simulink model "chooseTapB"  (Simulink 7.6)
settings: Solver=ode45  StartTime=0.0  StopTime=0.3  RelTol=1e-3
PreLoadFcn:
  | init
libraries: powerlib x19, dspsnks4 x5, fuzblock x3, factslib x1, powerlib_extras x1
settings Model: Creator=chix  LastModifiedBy=chix

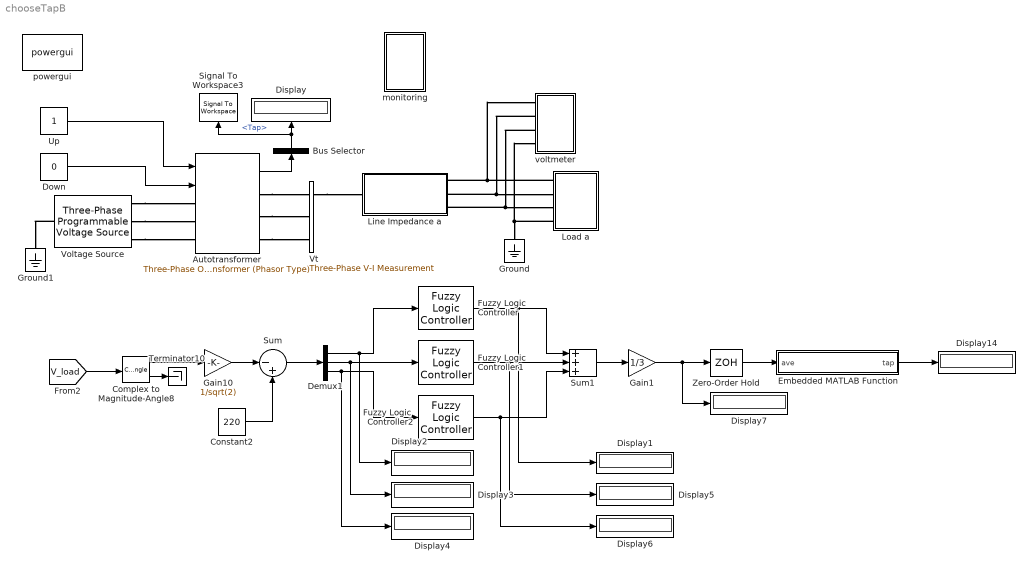
== system chooseTapB ==
  Autotransformer : factslib/Transformers/Three-Phase OLTC Regulating Transformer (Phasor Type)  DialogController=POWERSYS.PowerSysDialog  SystemSampleTime=-1  ShowParam=OLTC and Voltage Regulator parameters  PnomFnom="[200  60]"  Winding1=[220*sqrt(3) 0.00171 0.01714 ]  Winding1Connection=Yg  Winding2="[215*sqrt(3)   0.00094 0.01654 ]"  Winding2Connection=Yg  WindingTap=[ 0.00187 0.00142]  RmXm=[18.16805 1040.85906]  TapOnWinding=Winding 2  dU=3/215  TapMinMax="[ 0  4]"  InitialTap=2  TapSelectionTime=0.001  ExternalControl=on  RegulatorOn=on  Regulator=[1.0233 0.007 1]  Iw2_init="[0   0]"
  Bus Selector : BusSelector  OutputSignals=Tap
  Complex to Magnitude-Angle8 : ComplexToMagnitudeAngle
  Constant2 : Constant  Value=220
  Demux1 : Demux  Outputs=3
  Display{,1..7,14} (9 alike) : Display
  Down : Constant  Value=0
  Embedded MATLAB Function : Stateflow chart  TreatAsAtomicUnit=on
  Fuzzy Logic  Controller : fuzblock/Fuzzy Logic  Controller  SystemSampleTime=-1  fis='dataGather_w_con_1input_1.fis'
  Fuzzy Logic  Controller1 : fuzblock/Fuzzy Logic  Controller  SystemSampleTime=-1  fis='dataGather_w_con_1input_2.fis'
  Fuzzy Logic  Controller2 : fuzblock/Fuzzy Logic  Controller  SystemSampleTime=-1  fis='dataGather_w_con_1input_3.fis'
  Gain1 : Gain  Gain=1/3
  Gain10 : Gain  Gain=1/sqrt(2)
  Ground : powerlib/Elements/Ground  DialogController=POWERSYS.PowerSysDialog  PhysicalDomain=powersysdomain  SubClassName=unknown  LeftPortType=p1  RightPortType=p1  LConnTagsString=a
  Ground1 : powerlib/Elements/Ground  DialogController=POWERSYS.PowerSysDialog  PhysicalDomain=powersysdomain  SubClassName=unknown  LeftPortType=p1  RightPortType=p1  LConnTagsString=a
  Line Impedance a : Subsystem
  Load a : Subsystem
  Signal To Workspace3 : dspsnks4/Signal To Workspace  SystemSampleTime=-1  VariableName=tap  FrameMode=Concatenate frames (2-D array)
      settings: MaxDataPoints=1  FixptAsFi=off
  Sum : Sum  Inputs=|-+
  Sum1 : Sum  Inputs=+++
  Terminator10 : Terminator
  Up : Constant
  Voltage Source : powerlib/Electrical Sources/Three-Phase Programmable Voltage Source  DialogController=POWERSYS.PowerSysDialog  SystemSampleTime=-1  PositiveSequence="[220*sqrt(3)  0 60]"  VariationEntity=None  VariationType=Step  VariationStep=0.5  VariationRate=10  VariationMagnitude=0.3  VariationFrequency=2  VariationTiming=[1 2]  VariationPhaseA=off  Amplitudes=[1 0.8 1.2 1.0]  TimeValues=[0 0.1 0.15 0.2]  HarmonicGeneration=off  HarmonicA=[3 0.2 -25 0]  HarmonicB=[2 0.15 35 2]  Timing="[0.05  3]"
  Vt : powerlib/Measurements/Three-Phase V-I Measurement  DialogController=POWERSYS.PowerSysDialog  SystemSampleTime=-1  VoltageMeasurement=phase-to-ground  SetLabelV=on  LabelV=Vabc_xmer  Vpu=off  VpuLL=off  CurrentMeasurement=no  SetLabelI=off  LabelI=Iabc  Ipu=off  Pbase=100e6  Vbase=220  OutputType=Magnitude  PhasorSimulation=on  PSBequivalent=0
  Zero-Order Hold : ZeroOrderHold  SampleTime=0.011
  monitoring : Subsystem
  powergui : powerlib/powergui  Priority=1  SystemSampleTime=-1  SimulationMode=Phasor  SampleTime=50e-6  frequency=60  SPID=off  DisableSnubberDevices=off  DisableRonSwitches=off  DisableVfSwitches=off  SwTol=0  Interpol=off  frequencyindice=60  echomessages=off  HookPort=off  DisplayEquations=off  FunctionMessages=off  EnableUseOfTLC=off  x0status=blocks  RestoreLinks=warning  ResistiveCurrentMeasurement=off  Ylog=off  Xlog=on  ShowGrid=off  save=off  variable=ZData  ZoomFFT=off  StartTime=0.0  cycles=1  DisplayStyle=1  FreqAxis=off  MaxFrequency=1000  frequencyindicesteady=1  display=off  methode=off
  voltmeter : Subsystem
  wires:
  Bus Selector/1 -> Display/1, Signal To Workspace3/1  "<Tap>"
  Autotransformer/1 -> Bus Selector/1
  Complex to Magnitude-Angle8/1 -> Gain10/1
  [V_load] -> Complex to Magnitude-Angle8/1
  Gain10/1 -> Sum/1
  Constant2/1 -> Sum/2
  Sum/1 -> Demux1/1
  Demux1/1 -> Display2/1, Fuzzy Logic  Controller/1
  Demux1/3 -> Display4/1, Fuzzy Logic  Controller2/1
  Complex to Magnitude-Angle8/2 -> Terminator10/1
  Demux1/2 -> Display3/1, Fuzzy Logic  Controller1/1
  Fuzzy Logic  Controller/1 -> Display1/1, Sum1/1
  Fuzzy Logic  Controller1/1 -> Display5/1, Sum1/2
  Fuzzy Logic  Controller2/1 -> Display6/1, Sum1/3
  Sum1/1 -> Gain1/1
  Zero-Order Hold/1 -> Embedded MATLAB Function/1(ave)
  Embedded MATLAB Function/1(tap) -> Display14/1
  Gain1/1 -> Zero-Order Hold/1, Display7/1
  Down/1 -> Autotransformer/2
  Up/1 -> Autotransformer/1
  connections:
  Voltage Source/LConn1 -- Ground1/LConn1
  Voltage Source/RConn1 -- Autotransformer/LConn1
  Voltage Source/RConn2 -- Autotransformer/LConn2
  Voltage Source/RConn3 -- Autotransformer/LConn3
  Autotransformer/RConn3 -- Vt/LConn3
  Autotransformer/RConn2 -- Vt/LConn2
  Autotransformer/RConn1 -- Vt/LConn1
  Vt/RConn1 -- Line Impedance a/LConn1
  Load a/LConn4 -- Ground/LConn1 -- voltmeter/LConn4
  voltmeter/LConn3 -- Line Impedance a/RConn3 -- Load a/LConn3
  voltmeter/LConn2 -- Line Impedance a/RConn2 -- Load a/LConn2
  Load a/LConn1 -- Line Impedance a/RConn1 -- voltmeter/LConn1

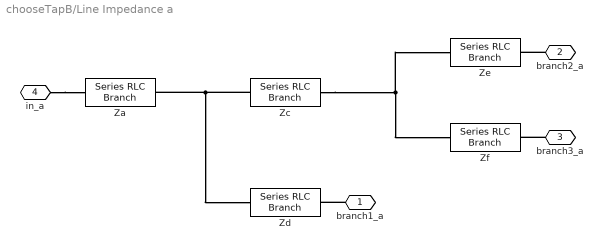
== system chooseTapB/Line Impedance a ==
  Za : powerlib/Elements/Series RLC Branch  DialogController=POWERSYS.PowerSysDialog  PhysicalDomain=powersysdomain  SubClassName=unknown  LeftPortType=p1  RightPortType=p1  LConnTagsString=__new0  RConnTagsString=__new0  BranchType=RL  Resistance=0.014  Inductance=0.0113e-3  SetiL0=off  InitialCurrent=0  Capacitance=1e-6  Setx0=off  InitialVoltage=0  Measurements=None
  Zc : powerlib/Elements/Series RLC Branch  DialogController=POWERSYS.PowerSysDialog  PhysicalDomain=powersysdomain  SubClassName=unknown  LeftPortType=p1  RightPortType=p1  LConnTagsString=__new0  RConnTagsString=__new0  BranchType=RL  Resistance=0.013  Inductance=0.0102e-3  SetiL0=off  InitialCurrent=0  Capacitance=1e-6  Setx0=off  InitialVoltage=0  Measurements=None
  Zd : powerlib/Elements/Series RLC Branch  DialogController=POWERSYS.PowerSysDialog  PhysicalDomain=powersysdomain  SubClassName=unknown  LeftPortType=p1  RightPortType=p1  LConnTagsString=__new0  RConnTagsString=__new0  BranchType=RL  Resistance=11  Inductance=47e-3  SetiL0=off  InitialCurrent=0  Capacitance=1e-6  Setx0=off  InitialVoltage=0  Measurements=None
  Ze : powerlib/Elements/Series RLC Branch  DialogController=POWERSYS.PowerSysDialog  PhysicalDomain=powersysdomain  SubClassName=unknown  LeftPortType=p1  RightPortType=p1  LConnTagsString=__new0  RConnTagsString=__new0  BranchType=RL  Resistance=1  Inductance=47e-3  SetiL0=off  InitialCurrent=0  Capacitance=1e-6  Setx0=off  InitialVoltage=0  Measurements=None
  Zf : powerlib/Elements/Series RLC Branch  DialogController=POWERSYS.PowerSysDialog  PhysicalDomain=powersysdomain  SubClassName=unknown  LeftPortType=p1  RightPortType=p1  LConnTagsString=__new0  RConnTagsString=__new0  BranchType=RL  Resistance=4.7  Inductance=21.5e-3  SetiL0=off  InitialCurrent=0  Capacitance=1e-6  Setx0=off  InitialVoltage=0  Measurements=None
  branch1_a : PMIOPort  Port=1  Side=Right
  branch2_a : PMIOPort  Port=2  Side=Right
  branch3_a : PMIOPort  Port=3  Side=Right
  in_a : PMIOPort  Port=4  Side=Left
  connections:
  Za/RConn1 -- Zc/LConn1 -- Zd/LConn1
  Zc/RConn1 -- Ze/LConn1 -- Zf/LConn1
  branch2_a/RConn1 -- Ze/RConn1
  in_a/RConn1 -- Za/LConn1
  branch3_a/RConn1 -- Zf/RConn1
  branch1_a/RConn1 -- Zd/RConn1

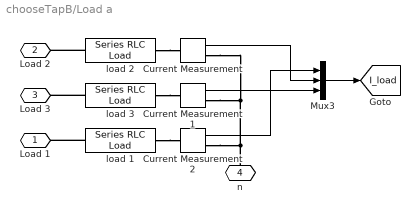
== system chooseTapB/Load a ==
  Current Measurement : powerlib/Measurements/Current Measurement  DialogController=POWERSYS.PowerSysDialog  SystemSampleTime=-1  PhasorSimulation=on  OutputType=Complex  PSBequivalent=0
  Current Measurement1 : powerlib/Measurements/Current Measurement  DialogController=POWERSYS.PowerSysDialog  SystemSampleTime=-1  PhasorSimulation=on  OutputType=Complex  PSBequivalent=0
  Current Measurement2 : powerlib/Measurements/Current Measurement  DialogController=POWERSYS.PowerSysDialog  SystemSampleTime=-1  PhasorSimulation=on  OutputType=Complex  PSBequivalent=0
  Mux3 : Mux  Inputs=3
  load 1 : powerlib/Elements/Series RLC Load  DialogController=POWERSYS.PowerSysDialog  PhysicalDomain=powersysdomain  SubClassName=unknown  LeftPortType=p1  RightPortType=p1  LConnTagsString=a  RConnTagsString=__new0  NominalVoltage=220  NominalFrequency=60  ActivePower=pow1  InductivePower=ql1  CapacitivePower=qc1  Setx0=off  InitialVoltage=0  SetiL0=off  InitialCurrent=0  Measurements=None
  load 2 : powerlib/Elements/Series RLC Load  DialogController=POWERSYS.PowerSysDialog  PhysicalDomain=powersysdomain  SubClassName=unknown  LeftPortType=p1  RightPortType=p1  LConnTagsString=a  RConnTagsString=__new0  NominalVoltage=220  NominalFrequency=60  ActivePower=pow2  InductivePower=ql2  CapacitivePower=qc2  Setx0=off  InitialVoltage=0  SetiL0=off  InitialCurrent=0  Measurements=None
  load 3 : powerlib/Elements/Series RLC Load  DialogController=POWERSYS.PowerSysDialog  PhysicalDomain=powersysdomain  SubClassName=unknown  LeftPortType=p1  RightPortType=p1  LConnTagsString=a  RConnTagsString=__new0  NominalVoltage=220  NominalFrequency=60  ActivePower=pow3  InductivePower=ql3  CapacitivePower=qc3  Setx0=off  InitialVoltage=0  SetiL0=off  InitialCurrent=0  Measurements=None
  Load 1 : PMIOPort  Port=1  Side=Left
  Load 2 : PMIOPort  Port=2  Side=Left
  Load 3 : PMIOPort  Port=3  Side=Left
  n : PMIOPort  Port=4  Side=Left
  tag scope: I_load=global
  wires:
  Mux3/1 -> [I_load]
  Current Measurement/1 -> Mux3/2
  Current Measurement1/1 -> Mux3/3
  Current Measurement2/1 -> Mux3/1
  connections:
  load 2/LConn1 -- Load 2/RConn1
  load 3/LConn1 -- Load 3/RConn1
  load 1/LConn1 -- Load 1/RConn1
  load 2/RConn1 -- Current Measurement/LConn1
  load 3/RConn1 -- Current Measurement1/LConn1
  load 1/RConn1 -- Current Measurement2/LConn1
  n/RConn1 -- Current Measurement/RConn1 -- Current Measurement1/RConn1 -- Current Measurement2/RConn1

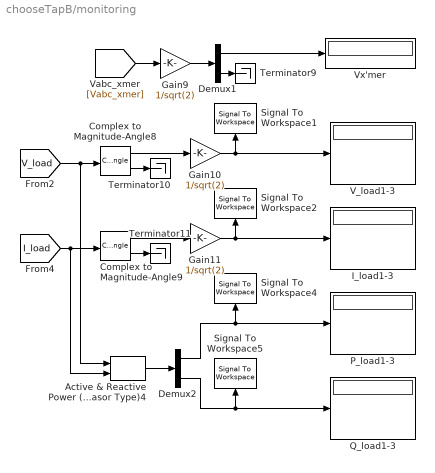
== system chooseTapB/monitoring ==
  Active & Reactive Power (Phasor Type)4 : powerlib_extras/Phasor Library/Active & Reactive Power (Phasor Type)  DialogController=POWERSYS.PowerSysDialog  SystemSampleTime=-1
  Complex to Magnitude-Angle8 : ComplexToMagnitudeAngle
  Complex to Magnitude-Angle9 : ComplexToMagnitudeAngle
  Demux1 : Demux  Outputs=[1 2]
  Demux2 : Demux  Outputs=[3 3]
  Gain10 : Gain  Gain=1/sqrt(2)
  Gain11 : Gain  Gain=1/sqrt(2)
  Gain9 : Gain  Gain=1/sqrt(2)
  I_load1-3 : Display
  P_load1-3 : Display
  Q_load1-3 : Display
  Signal To Workspace1 : dspsnks4/Signal To Workspace  SystemSampleTime=-1  VariableName=vload  FrameMode=Concatenate frames (2-D array)
      settings: MaxDataPoints=1  FixptAsFi=off
  Signal To Workspace2 : dspsnks4/Signal To Workspace  SystemSampleTime=-1  VariableName=iload  FrameMode=Concatenate frames (2-D array)
      settings: MaxDataPoints=1  FixptAsFi=off
  Signal To Workspace4 : dspsnks4/Signal To Workspace  SystemSampleTime=-1  VariableName=pload  FrameMode=Concatenate frames (2-D array)
      settings: MaxDataPoints=1  FixptAsFi=off
  Signal To Workspace5 : dspsnks4/Signal To Workspace  SystemSampleTime=-1  VariableName=qload  FrameMode=Concatenate frames (2-D array)
      settings: MaxDataPoints=1  FixptAsFi=off
  Terminator10 : Terminator
  Terminator11 : Terminator
  Terminator9 : Terminator
  V_load1-3 : Display
  Vx'mer : Display
  wires:
  [Vabc_xmer] -> Gain9/1
  Gain9/1 -> Demux1/1
  Demux1/1 -> Vx'mer/1
  Demux1/2 -> Terminator9/1
  Complex to Magnitude-Angle8/1 -> Gain10/1
  Complex to Magnitude-Angle8/2 -> Terminator10/1
  [V_load] -> Complex to Magnitude-Angle8/1, Active & Reactive Power (Phasor Type)4/1
  Gain10/1 -> V_load1-3/1, Signal To Workspace1/1
  Complex to Magnitude-Angle9/1 -> Gain11/1
  Complex to Magnitude-Angle9/2 -> Terminator11/1
  [I_load] -> Complex to Magnitude-Angle9/1, Active & Reactive Power (Phasor Type)4/2
  Gain11/1 -> I_load1-3/1, Signal To Workspace2/1
  Active & Reactive Power (Phasor Type)4/1 -> Demux2/1
  Demux2/1 -> P_load1-3/1, Signal To Workspace4/1
  Demux2/2 -> Q_load1-3/1, Signal To Workspace5/1

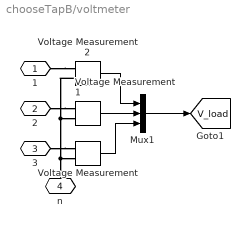
== system chooseTapB/voltmeter ==
  Mux1 : Mux  Inputs=3
  Voltage Measurement : powerlib/Measurements/Voltage Measurement  DialogController=POWERSYS.PowerSysDialog  SystemSampleTime=-1  PhasorSimulation=on  OutputType=Complex  PSBequivalent=0
  Voltage Measurement1 : powerlib/Measurements/Voltage Measurement  DialogController=POWERSYS.PowerSysDialog  SystemSampleTime=-1  PhasorSimulation=on  OutputType=Complex  PSBequivalent=0
  Voltage Measurement2 : powerlib/Measurements/Voltage Measurement  DialogController=POWERSYS.PowerSysDialog  SystemSampleTime=-1  PhasorSimulation=on  OutputType=Complex  PSBequivalent=0
  1 : PMIOPort  Port=1  Side=Left
  2 : PMIOPort  Port=2  Side=Left
  3 : PMIOPort  Port=3  Side=Left
  n : PMIOPort  Port=4  Side=Left
  tag scope: V_load=global
  wires:
  Mux1/1 -> [V_load]
  Voltage Measurement1/1 -> Mux1/2
  Voltage Measurement2/1 -> Mux1/1
  Voltage Measurement/1 -> Mux1/3
  connections:
  Voltage Measurement1/LConn2 -- Voltage Measurement2/LConn2 -- Voltage Measurement/LConn2 -- n/RConn1
  1/RConn1 -- Voltage Measurement2/LConn1
  2/RConn1 -- Voltage Measurement1/LConn1
  3/RConn1 -- Voltage Measurement/LConn1

== matlab function Embedded MATLAB Function ==
  data: ave input double; tap output double
function tap=chooseTap(ave)
%#eml

if ave>=60
    tap=4;
elseif ave<60&&ave>20
    tap=3;
elseif ave<=20&&ave>=-20
    tap=2;
elseif ave<-20&&ave>-60
    tap=1;
else
    tap=0;
end
